simulink model "gm_sampleModel1839_4_sub"  (R2023a)
settings: Solver=VariableStepAuto  StartTime=0.0  StopTime=10.0  RelTol=1e-3
libraries: simulink x1
settings Model: Creator=user1  LastModifiedBy=user1
settings OptimizationCC: BlockReduction=off  ConditionallyExecuteInputs=off
settings DebuggingCC: InheritedTsInSrcMsg=none

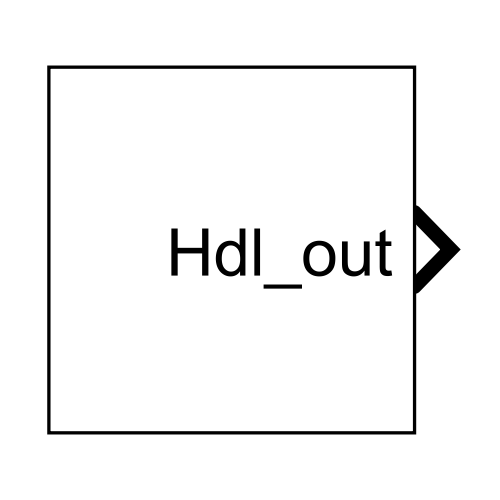
[thumbnail: Simulink's stored preview of the top-level diagram]
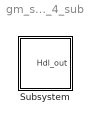
== system gm_sampleModel1839_4_sub ==
  Subsystem : Subsystem

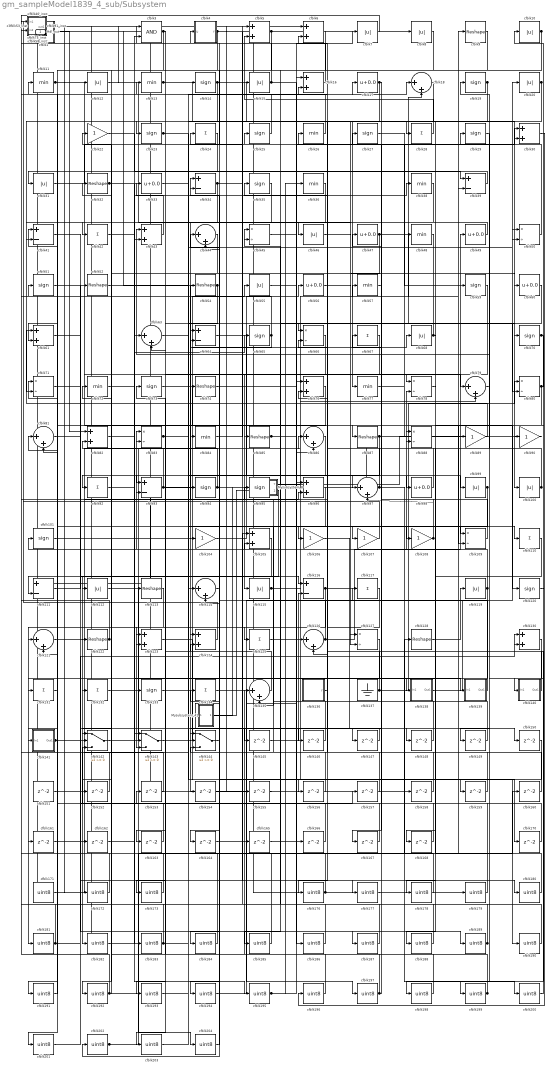
== system gm_sampleModel1839_4_sub/Subsystem ==
  Mysubsystem_41 : Subsystem
  Mysubsystem_8 : Subsystem
  cfblk1 : Subsystem  mask(Detect Rise Positive){vinit=double(0), InputProcessing=Elements as channels (sample based), OutDataTypeStr=uint8}
      mask prompts: vinit "Simulink:masks:InitialCondition_MP"; InputProcessing "Simulink:masks:InputProcessing_MP"; OutDataTypeStr "Simulink:masks:OutputDataType_MP"
      mask help: Simulink:masks:DetectRisePositive_MD
      mask init:
      | InputProcessing = 'Elements as channels (sample based)';
      | OutDataTypeStr = 'uint8';
      | vinit = double(0);
      mask TypeOptions InputProcessing: Simulink:masks:ColumnsAsChannelsFrameBased | Simulink:masks:ElementsAsChannelsSampleBased
      mask TypeOptions OutDataTypeStr: Simulink:masks:uint8 | Simulink:masks:boolean
      mask Display: fprintf('U > 0\n&  NOT\nU/z > 0')
  cfblk{7..8,10,12,15,20,31,46,55,68,99..100,112,115,119} (15 alike) : Abs  OutDataTypeStr=uint8  SaturateOnIntegerOverflow=off
  cfblk{14,19,23,25,27,29,35,51,59,65,70,73,94..95,101,120,133} (17 alike) : Signum
  cfblk102_inst : Subsystem
  cfblk{22,89..90,104,106..108} (7 alike) : Gain  OutDataTypeStr=uint8
  cfblk{5..6,16,30,43,61,76,82,96,105,123..124,130} (13 alike) : Sum  OutDataTypeStr=uint8
  cfblk{45,50,66,71,78,80,83,88,109,127} (10 alike) : Product  Inputs=*/  OutDataTypeStr=uint8  RndMeth=Zero  SaturateOnIntegerOverflow=on
  cfblk{11,13,26,36,38,48,57,72,77,84} (10 alike) : MinMax  OutDataTypeStr=uint8
  cfblk{24,28,42,67,92,110,117,125,131..132,134} (11 alike) : Sum  Inputs=+  OutDataTypeStr=uint8
  cfblk{34,39,41,64,93,111,116} (7 alike) : Sum  Inputs=+-  OutDataTypeStr=uint8
  cfblk{9,32,52,54,74,85,87,113,122,128} (10 alike) : Reshape
  cfblk{18,44,63,79,81,86,97,114,121,126,135} (11 alike) : Sum  Inputs=|++  OutDataTypeStr=uint8
  cfblk118_inst : Subsystem
  cfblk129_inst : Subsystem
  cfblk136 : Subsystem  mask(Counter Free-Running){NumBits=double(16), tsamp=double(-1)}
      mask prompts: NumBits "Simulink:masks:NumberOfBits_MP"; tsamp "Simulink:masks:SampleTime_MP"
      mask help: Simulink:masks:CounterFreeRunning_MD
  cfblk137 : Ground
  cfblk138 : Subsystem
  cfblk139 : Subsystem
  cfblk140 : Subsystem
  cfblk141 : Subsystem
  cfblk142 : Switch  OutDataTypeStr=uint8  SaturateOnIntegerOverflow=off  InputSameDT=off
  cfblk143 : Switch  OutDataTypeStr=uint8  SaturateOnIntegerOverflow=off  InputSameDT=off
  cfblk144 : Switch  OutDataTypeStr=uint8  SaturateOnIntegerOverflow=off  InputSameDT=off
  cfblk{145..168,170} (25 alike) : Delay  SampleTime=1
  cfblk{17,33,47,49,56,60,98} (7 alike) : Bias  Bias=0.0  SaturateOnIntegerOverflow=off
  cfblk{171..173,176..204} (32 alike) : DataTypeConversion  OutDataTypeStr=uint8  SaturateOnIntegerOverflow=off  RndMeth=Floor
  cfblk21_inst : Subsystem
  cfblk3 : Logic  AllPortsSameDT=off  OutDataTypeStr=boolean
  cfblk37_inst : Subsystem
  cfblk4 : Subsystem  mask(Detect Rise Nonnegative){vinit=double(0), InputProcessing=Elements as channels (sample based), OutDataTypeStr=uint8}
      mask prompts: vinit "Simulink:masks:InitialCondition_MP"; InputProcessing "Simulink:masks:InputProcessing_MP"; OutDataTypeStr "Simulink:masks:OutputDataType_MP"
      mask help: Simulink:masks:DetectRiseNonnegative_MD
      mask init:
      | InputProcessing = 'Elements as channels (sample based)';
      | OutDataTypeStr = 'uint8';
      | vinit = double(0);
      mask TypeOptions InputProcessing: Simulink:masks:ColumnsAsChannelsFrameBased | Simulink:masks:ElementsAsChannelsSampleBased
      mask TypeOptions OutDataTypeStr: Simulink:masks:uint8 | Simulink:masks:boolean
      mask Display: fprintf('U >= 0\n&  NOT\nU/z >= 0')
  cfblk40_inst : Subsystem
  cfblk53_inst : Subsystem
  cfblk58_inst : Subsystem
  cfblk75_inst : Subsystem
  cfblk91_inst : Subsystem
  Hdl_out : Outport  OutDataTypeStr=uint8  SampleTime=1
  wires:
  Mysubsystem_41/1(Out1) -> Mysubsystem_8/2(In2)
  Mysubsystem_8/1(Y) -> cfblk79/2
  Mysubsystem_8/2(Out2) -> cfblk111/2
  cfblk1/1(Y) -> cfblk82/1
  cfblk10/1 -> cfblk63/2, cfblk201/1
  cfblk100/1 -> cfblk43/1, cfblk16/2
  cfblk101/1 -> cfblk107/1
  cfblk102_inst/1(out1) -> cfblk6/1
  cfblk104/1 -> cfblk56/1
  cfblk105/1 -> cfblk182/1
  cfblk106/1 -> cfblk148/1
  cfblk107/1 -> cfblk102_inst/1(in1)
  cfblk108/1 -> cfblk97/2, cfblk24/1
  cfblk109/1 -> cfblk25/1
  cfblk11/1 -> cfblk115/1, cfblk78/1
  cfblk110/1 -> cfblk156/1
  cfblk111/1 -> cfblk52/1
  cfblk112/1 -> cfblk204/1
  cfblk113/1 -> cfblk181/1
  cfblk114/1 -> cfblk202/1
  cfblk115/1 -> cfblk18/2, cfblk170/1
  cfblk116/1 -> cfblk49/1, cfblk143/3
  cfblk117/1 -> cfblk176/1
  cfblk118_inst/1(out1) -> cfblk171/1
  cfblk119/1 -> cfblk83/1, cfblk161/1
  cfblk12/1 -> cfblk154/1
  cfblk120/1 -> cfblk198/1
  cfblk121/1 -> cfblk96/2
  cfblk122/1 -> cfblk41/1, cfblk129_inst/1(in1)
  cfblk123/1 -> cfblk190/1
  cfblk124/1 -> cfblk75_inst/2(in2)
  cfblk125/1 -> cfblk166/1
  cfblk126/1 -> cfblk101/1, cfblk78/2
  cfblk127/1 -> cfblk163/1
  cfblk128/1 -> cfblk119/1
  cfblk129_inst/1(out1) -> cfblk179/1, cfblk12/1
  cfblk13/1 -> cfblk100/1, cfblk127/2
  cfblk130/1 -> cfblk199/1
  cfblk131/1 -> cfblk71/1
  cfblk132/1 -> cfblk63/1
  cfblk133/1 -> cfblk55/1
  cfblk134/1 -> cfblk197/1
  cfblk135/1 -> cfblk73/1
  cfblk136/1(y) -> cfblk26/1
  cfblk137/1 -> cfblk95/1, cfblk80/1
  cfblk138/1(Out1) -> cfblk20/1
  cfblk139/1(Out1) -> cfblk51/1
  cfblk14/1 -> cfblk23/1, cfblk77/1
  cfblk140/1(Out1) -> cfblk35/1
  cfblk141/1(Out1) -> cfblk54/1, cfblk57/1
  cfblk142/1 -> cfblk9/1
  cfblk143/1 -> cfblk68/1
  cfblk144/1 -> cfblk34/1
  cfblk145/1 -> cfblk116/2
  cfblk146/1 -> cfblk64/1
  cfblk147/1 -> cfblk144/2
  cfblk148/1 -> cfblk66/2
  cfblk149/1 -> cfblk102_inst/2(in2)
  cfblk15/1 -> cfblk99/1, cfblk53_inst/2(in2)
  cfblk150/1 -> cfblk184/1
  cfblk151/1 -> cfblk96/1
  cfblk152/1 -> cfblk121/2
  cfblk153/1 -> cfblk37_inst/1(in1)
  cfblk154/1 -> cfblk50/2
  cfblk155/1 -> cfblk1/1(U)
  cfblk156/1 -> cfblk34/2
  cfblk157/1 -> cfblk76/2
  cfblk158/1 -> cfblk105/2
  cfblk159/1 -> cfblk126/2
  cfblk16/1 -> cfblk3/1
  cfblk160/1 -> cfblk6/2
  cfblk161/1 -> cfblk3/2
  cfblk162/1 -> cfblk143/1
  cfblk163/1 -> cfblk142/3
  cfblk164/1 -> cfblk135/1
  cfblk165/1 -> cfblk30/1
  cfblk166/1 -> cfblk82/2
  cfblk167/1 -> cfblk142/2
  cfblk168/1 -> cfblk144/3
  cfblk17/1 -> cfblk147/1, cfblk146/1
  cfblk170/1 -> cfblk11/1
  cfblk171/1 -> cfblk94/1
  cfblk172/1 -> cfblk118_inst/1(in1)
  cfblk173/1 -> cfblk118_inst/2(in2)
  cfblk176/1 -> cfblk58_inst/2(in2), cfblk44/1
  cfblk177/1 -> cfblk117/1
  cfblk178/1 -> cfblk153/1
  cfblk179/1 -> cfblk88/1
  cfblk18/1 -> cfblk124/1
  cfblk180/1 -> cfblk88/2
  cfblk181/1 -> cfblk91_inst/1(in1), cfblk187/1, cfblk157/1
  cfblk182/1 -> cfblk113/1
  cfblk183/1 -> cfblk53_inst/1(in1), cfblk50/1
  cfblk184/1 -> cfblk21_inst/1(in1)
  cfblk185/1 -> cfblk21_inst/2(in2)
  cfblk186/1 -> cfblk37_inst/2(in2)
  cfblk187/1 -> cfblk45/1
  cfblk188/1 -> cfblk45/2
  cfblk189/1 -> cfblk129_inst/2(in2), cfblk105/1
  cfblk19/1 -> cfblk194/1, cfblk84/1
  cfblk190/1 -> cfblk81/1
  cfblk191/1 -> cfblk81/2
  cfblk192/1 -> cfblk40_inst/2(in2), cfblk39/2, cfblk22/1
  cfblk193/1 -> cfblk86/1
  cfblk194/1 -> cfblk86/2
  cfblk195/1 -> cfblk76/1, cfblk36/1
  cfblk196/1 -> cfblk72/1
  cfblk197/1 -> cfblk47/1, cfblk124/2
  cfblk198/1 -> cfblk134/1
  cfblk199/1 -> cfblk93/2, cfblk155/1
  cfblk20/1 -> cfblk188/1, cfblk71/2, cfblk141/1(In1)
  cfblk200/1 -> cfblk130/1
  cfblk201/1 -> cfblk130/2
  cfblk202/1 -> cfblk128/1, cfblk160/1
  cfblk203/1 -> cfblk114/1
  cfblk204/1 -> cfblk114/2
  cfblk21_inst/1(out1) -> cfblk183/1
  cfblk22/1 -> cfblk39/1
  cfblk23/1 -> cfblk109/1, cfblk28/1
  cfblk24/1 -> cfblk112/1
  cfblk25/1 -> cfblk13/1
  cfblk26/1 -> cfblk58_inst/1(in1)
  cfblk27/1 -> cfblk59/1
  cfblk28/1 -> cfblk5/2
  cfblk29/1 -> cfblk149/1
  cfblk3/1 -> cfblk61/2, cfblk203/1
  cfblk30/1 -> cfblk196/1
  cfblk31/1 -> cfblk15/1
  cfblk32/1 -> cfblk43/2, cfblk127/1
  cfblk33/1 -> cfblk97/1
  cfblk34/1 -> cfblk79/1, cfblk193/1, cfblk143/2
  cfblk35/1 -> cfblk131/1
  cfblk36/1 -> cfblk41/2
  cfblk37_inst/1(out1) -> cfblk8/1, cfblk133/1
  cfblk38/1 -> cfblk132/1
  cfblk39/1 -> cfblk31/1
  cfblk4/1(Y) -> cfblk180/1, cfblk173/1, cfblk92/1, cfblk42/1
  cfblk40_inst/1(out1) -> cfblk75_inst/1(in1)
  cfblk41/1 -> cfblk150/1
  cfblk42/1 -> cfblk38/1
  cfblk43/1 -> cfblk33/1
  cfblk44/1 -> cfblk93/1
  cfblk45/1 -> cfblk186/1
  cfblk46/1 -> cfblk60/1
  cfblk47/1 -> cfblk80/2, cfblk152/1
  cfblk48/1 -> cfblk125/1
  cfblk49/1 -> cfblk46/1
  cfblk5/1 -> cfblk165/1, cfblk164/1
  cfblk50/1 -> cfblk4/1(U)
  cfblk51/1 -> cfblk116/1
  cfblk52/1 -> cfblk70/1
  cfblk53_inst/1(out1) -> cfblk172/1
  cfblk54/1 -> cfblk123/2, Hdl_out/1
  cfblk55/1 -> cfblk7/1
  cfblk56/1 -> cfblk98/1
  cfblk57/1 -> cfblk167/1
  cfblk58_inst/1(out1) -> cfblk14/1
  cfblk59/1 -> cfblk123/1
  cfblk6/1 -> cfblk144/1
  cfblk60/1 -> cfblk145/1
  cfblk61/1 -> cfblk162/1
  cfblk63/1 -> cfblk18/1
  cfblk64/1 -> cfblk126/1
  cfblk65/1 -> cfblk91_inst/2(in2), cfblk64/2
  cfblk66/1 -> cfblk85/1
  cfblk67/1 -> cfblk106/1
  cfblk68/1 -> cfblk66/1, cfblk168/1
  cfblk7/1 -> cfblk40_inst/1(in1)
  cfblk70/1 -> cfblk90/1, cfblk140/1(In1)
  cfblk71/1 -> cfblk177/1
  cfblk72/1 -> cfblk195/1
  cfblk73/1 -> cfblk120/1
  cfblk74/1 -> cfblk27/1
  cfblk75_inst/1(out1) -> cfblk151/1
  cfblk76/1 -> cfblk121/1
  cfblk77/1 -> cfblk48/1
  cfblk78/1 -> cfblk108/1
  cfblk79/1 -> cfblk19/1
  cfblk8/1 -> cfblk122/1
  cfblk80/1 -> cfblk10/1, cfblk109/2, cfblk138/1(In1)
  cfblk81/1 -> cfblk189/1
  cfblk82/1 -> cfblk65/1
  cfblk83/1 -> cfblk74/1, cfblk159/1
  cfblk84/1 -> cfblk5/1
  cfblk85/1 -> cfblk87/1, cfblk17/1
  cfblk86/1 -> cfblk192/1
  cfblk87/1 -> cfblk30/2, cfblk29/1, cfblk104/1
  cfblk88/1 -> cfblk178/1
  cfblk89/1 -> cfblk61/1
  cfblk9/1 -> cfblk185/1
  cfblk90/1 -> Mysubsystem_8/1(In1)
  cfblk91_inst/1(out1) -> cfblk158/1
  cfblk92/1 -> cfblk139/1(In1)
  cfblk93/1 -> cfblk83/2, cfblk110/1
  cfblk94/1 -> cfblk44/2, cfblk32/1
  cfblk95/1 -> cfblk111/1, cfblk89/1, Mysubsystem_41/1(In1)
  cfblk96/1 -> cfblk135/2
  cfblk97/1 -> cfblk200/1, cfblk16/1
  cfblk98/1 -> cfblk67/1
  cfblk99/1 -> cfblk191/1, cfblk142/1

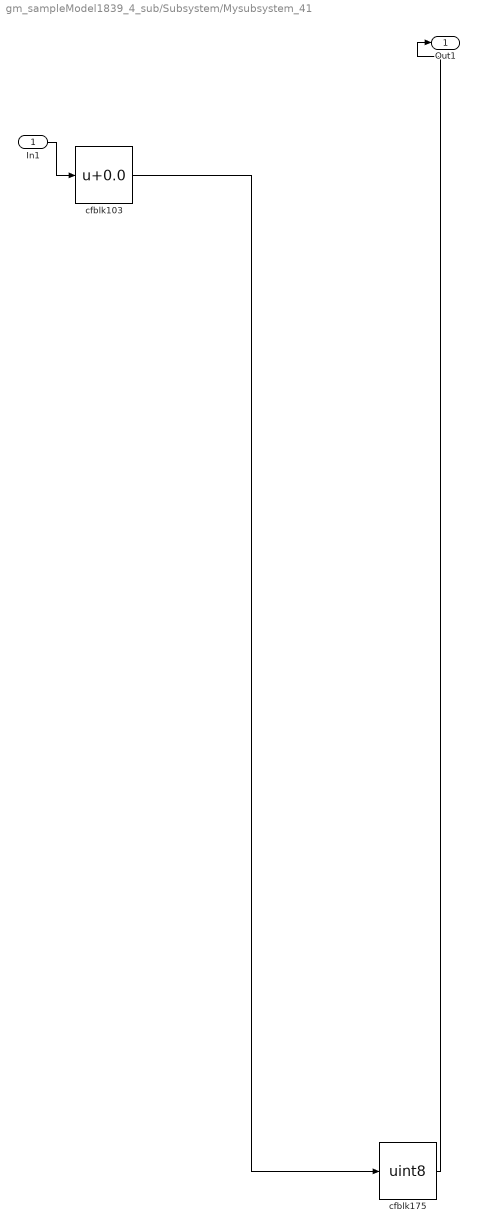
== system gm_sampleModel1839_4_sub/Subsystem/Mysubsystem_41 ==
  In1 : Inport  OutDataTypeStr=uint8  PortDimensions=1  SampleTime=1
  cfblk103 : Bias  Bias=0.0  SaturateOnIntegerOverflow=off
  cfblk175 : DataTypeConversion  OutDataTypeStr=uint8  SaturateOnIntegerOverflow=off  RndMeth=Floor
  Out1 : Outport  SampleTime=1
  wires:
  In1/1 -> cfblk103/1
  cfblk103/1 -> cfblk175/1
  cfblk175/1 -> Out1/1

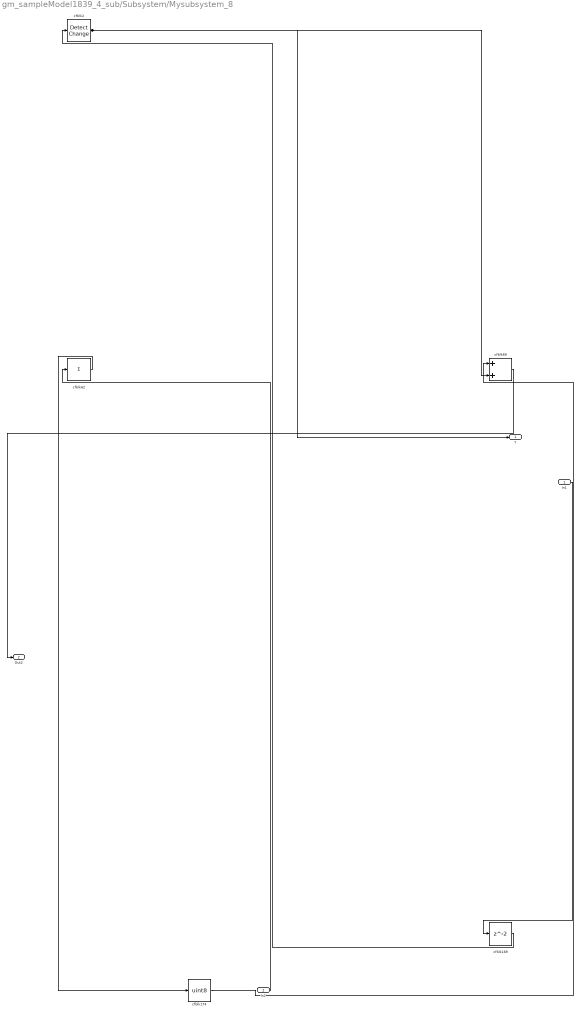
== system gm_sampleModel1839_4_sub/Subsystem/Mysubsystem_8 ==
  In1 : Inport  OutDataTypeStr=uint8  PortDimensions=1  SampleTime=1
  In2 : Inport  Port=2  OutDataTypeStr=uint8  PortDimensions=1  SampleTime=1
  cfblk169 : Delay  SampleTime=1
  cfblk174 : DataTypeConversion  OutDataTypeStr=uint8  SaturateOnIntegerOverflow=off  RndMeth=Floor
  cfblk2 : simulink/Logic and Bit Operations/Detect Change  vinit=0  OutDataTypeStr=boolean
      settings: LibrarySourceBlock=|
      | hdlsllib/Logic and Bit
      | Operations/Detect
      | Change
  cfblk62 : Sum  Inputs=+
  cfblk69 : Sum
  Y : Outport  SampleTime=1
  Out2 : Outport  Port=2  SampleTime=1
  wires:
  In1/1 -> cfblk169/1
  In2/1 -> cfblk62/1
  cfblk169/1 -> cfblk2/1
  cfblk174/1 -> cfblk69/1
  cfblk2/1 -> cfblk69/2, Y/1
  cfblk62/1 -> cfblk174/1
  cfblk69/1 -> Out2/1

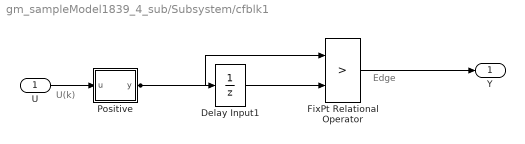
== system gm_sampleModel1839_4_sub/Subsystem/cfblk1 ==
  note: U(k)
  note: Edge
  U : Inport  OutDataTypeStr=uint8  SampleTime=1
  Delay Input1 : UnitDelay  Description=Store in Global RAM  DisableCoverage=on  InitialCondition=vinit  SampleTime=-1  HasFrameUpgradeWarning=on
  FixPt Relational Operator : RelationalOperator  Operator=>  OutDataTypeStr=fixdt(0, 8)  ZeroCross=off  InputSameDT=off
  Positive : Subsystem  mask(Compare To Zero){relop=>, OutDataTypeStr=boolean, ZeroCross=off}
      mask prompts: relop "Simulink:masks:Operator_MP"; OutDataTypeStr "Simulink:masks:OutputDataType_MP"; ZeroCross "Simulink:masks:EnableZerocrossingDetection_MP"
      mask help: Simulink:masks:CompareToZero_MD
      mask init:
      | OutDataTypeStr = 'boolean';
      | ZeroCross = 'off';
      | blkName = 'sampleModel1839_4_sub/Subsystem/cfblk1/Positive';
      | relop = '>';
      | setValue = 'boolean';
      mask TypeOptions relop: == | ~= | < | <= | >= | >
      mask TypeOptions OutDataTypeStr: Simulink:masks:uint8 | Simulink:masks:boolean
      mask Callback ZeroCross: sl('zeroCrossEnable', gcbh);
      mask Display: disp([relop,' 0'])
  Y : Outport  SampleTime=1
  wires:
  U/1 -> Positive/1(u)
  Delay Input1/1 -> FixPt Relational Operator/2
  FixPt Relational Operator/1 -> Y/1
  Positive/1(y) -> FixPt Relational Operator/1, Delay Input1/1

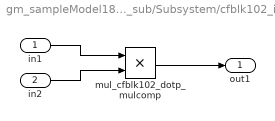
== system gm_sampleModel1839_4_sub/Subsystem/cfblk102_inst ==
  in1 : Inport  OutDataTypeStr=uint8  SampleTime=1
  in2 : Inport  Port=2  OutDataTypeStr=uint8  SampleTime=1
  mul_cfblk102_dotp_mulcomp : Product  Inputs=**  OutDataTypeStr=uint8  SampleTime=1
  out1 : Outport  OutDataTypeStr=uint8  SampleTime=1
  wires:
  in1/1 -> mul_cfblk102_dotp_mulcomp/1
  in2/1 -> mul_cfblk102_dotp_mulcomp/2
  mul_cfblk102_dotp_mulcomp/1 -> out1/1

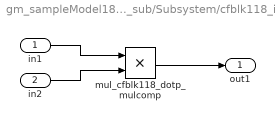
== system gm_sampleModel1839_4_sub/Subsystem/cfblk118_inst ==
  in1 : Inport  OutDataTypeStr=uint8  SampleTime=1
  in2 : Inport  Port=2  OutDataTypeStr=uint8  SampleTime=1
  mul_cfblk118_dotp_mulcomp : Product  Inputs=**  OutDataTypeStr=uint8  SampleTime=1
  out1 : Outport  OutDataTypeStr=uint8  SampleTime=1
  wires:
  in1/1 -> mul_cfblk118_dotp_mulcomp/1
  in2/1 -> mul_cfblk118_dotp_mulcomp/2
  mul_cfblk118_dotp_mulcomp/1 -> out1/1

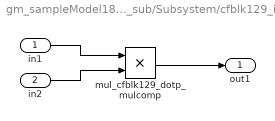
== system gm_sampleModel1839_4_sub/Subsystem/cfblk129_inst ==
  in1 : Inport  OutDataTypeStr=uint8  SampleTime=1
  in2 : Inport  Port=2  OutDataTypeStr=uint8  SampleTime=1
  mul_cfblk129_dotp_mulcomp : Product  Inputs=**  OutDataTypeStr=uint8  SampleTime=1
  out1 : Outport  OutDataTypeStr=uint8  SampleTime=1
  wires:
  in1/1 -> mul_cfblk129_dotp_mulcomp/1
  in2/1 -> mul_cfblk129_dotp_mulcomp/2
  mul_cfblk129_dotp_mulcomp/1 -> out1/1

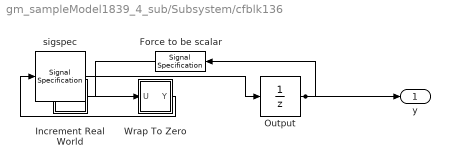
== system gm_sampleModel1839_4_sub/Subsystem/cfblk136 ==
  Force to be scalar : SignalSpecification  DisableCoverage=on  Dimensions=1
  Increment Real World : Subsystem  mask(Real World Value Increment){}
      mask help: Simulink:masks:RealWorldValueIncrement_MD
      mask Display: disp('V++')
  Output : UnitDelay  InitialCondition=0.0  SampleTime=tsamp  HasFrameUpgradeWarning=on
  Wrap To Zero : Subsystem  mask(Wrap To Zero){Threshold=double(65535)}
      mask prompts: Threshold "Simulink:masks:Threshold_MP"
      mask help: Simulink:masks:WrapToZero_MD
  sigspec : SignalSpecification  OutDataTypeStr=uint16  Dimensions=1
  y : Outport  SampleTime=1
  wires:
  Force to be scalar/1 -> Increment Real World/1(u)
  Increment Real World/1(y) -> Wrap To Zero/1(U)
  Output/1 -> Force to be scalar/1, y/1
  Wrap To Zero/1(Y) -> sigspec/1
  sigspec/1 -> Output/1

== system gm_sampleModel1839_4_sub/Subsystem/cfblk138 ==
  In1 : Inport  OutDataTypeStr=uint8  PortDimensions=1  SampleTime=1
  Out1 : Outport  SampleTime=1
  wires:
  In1/1 -> Out1/1

== system gm_sampleModel1839_4_sub/Subsystem/cfblk139 ==
  In1 : Inport  OutDataTypeStr=uint8  PortDimensions=1  SampleTime=1
  Out1 : Outport  SampleTime=1
  wires:
  In1/1 -> Out1/1

== system gm_sampleModel1839_4_sub/Subsystem/cfblk140 ==
  In1 : Inport  OutDataTypeStr=uint8  PortDimensions=1  SampleTime=1
  Out1 : Outport  SampleTime=1
  wires:
  In1/1 -> Out1/1

== system gm_sampleModel1839_4_sub/Subsystem/cfblk141 ==
  In1 : Inport  OutDataTypeStr=uint8  PortDimensions=1  SampleTime=1
  Out1 : Outport  SampleTime=1
  wires:
  In1/1 -> Out1/1

== system gm_sampleModel1839_4_sub/Subsystem/cfblk21_inst ==
  in1 : Inport  OutDataTypeStr=uint8  SampleTime=1
  in2 : Inport  Port=2  OutDataTypeStr=uint8  SampleTime=1
  mul_cfblk21_dotp_mulcomp : Product  Inputs=**  OutDataTypeStr=uint8  SampleTime=1
  out1 : Outport  OutDataTypeStr=uint8  SampleTime=1
  wires:
  in1/1 -> mul_cfblk21_dotp_mulcomp/1
  in2/1 -> mul_cfblk21_dotp_mulcomp/2
  mul_cfblk21_dotp_mulcomp/1 -> out1/1

== system gm_sampleModel1839_4_sub/Subsystem/cfblk37_inst ==
  in1 : Inport  OutDataTypeStr=uint8  SampleTime=1
  in2 : Inport  Port=2  OutDataTypeStr=uint8  SampleTime=1
  mul_cfblk37_dotp_mulcomp : Product  Inputs=**  OutDataTypeStr=uint8  SampleTime=1
  out1 : Outport  OutDataTypeStr=uint8  SampleTime=1
  wires:
  in1/1 -> mul_cfblk37_dotp_mulcomp/1
  in2/1 -> mul_cfblk37_dotp_mulcomp/2
  mul_cfblk37_dotp_mulcomp/1 -> out1/1

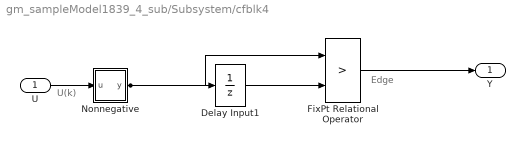
== system gm_sampleModel1839_4_sub/Subsystem/cfblk4 ==
  note: U(k)
  note: Edge
  U : Inport  OutDataTypeStr=uint8  SampleTime=1
  Delay Input1 : UnitDelay  Description=Store in Global RAM  DisableCoverage=on  InitialCondition=vinit  SampleTime=-1  HasFrameUpgradeWarning=on
  FixPt Relational Operator : RelationalOperator  Operator=>  OutDataTypeStr=fixdt(0, 8)  ZeroCross=off  InputSameDT=off
  Nonnegative : Subsystem  mask(Compare To Zero){relop=>=, OutDataTypeStr=boolean, ZeroCross=off}
      mask prompts: relop "Simulink:masks:Operator_MP"; OutDataTypeStr "Simulink:masks:OutputDataType_MP"; ZeroCross "Simulink:masks:EnableZerocrossingDetection_MP"
      mask help: Simulink:masks:CompareToZero_MD
      mask init:
      | OutDataTypeStr = 'boolean';
      | ZeroCross = 'off';
      | blkName = 'sampleModel1839_4_sub/Subsystem/cfblk4/Nonnegative';
      | relop = '>=';
      | setValue = 'boolean';
      mask TypeOptions relop: == | ~= | < | <= | >= | >
      mask TypeOptions OutDataTypeStr: Simulink:masks:uint8 | Simulink:masks:boolean
      mask Callback ZeroCross: sl('zeroCrossEnable', gcbh);
      mask Display: disp([relop,' 0'])
  Y : Outport  SampleTime=1
  wires:
  U/1 -> Nonnegative/1(u)
  Delay Input1/1 -> FixPt Relational Operator/2
  FixPt Relational Operator/1 -> Y/1
  Nonnegative/1(y) -> FixPt Relational Operator/1, Delay Input1/1

== system gm_sampleModel1839_4_sub/Subsystem/cfblk40_inst ==
  in1 : Inport  OutDataTypeStr=uint8  SampleTime=1
  in2 : Inport  Port=2  OutDataTypeStr=uint8  SampleTime=1
  mul_cfblk40_dotp_mulcomp : Product  Inputs=**  OutDataTypeStr=uint8  SampleTime=1
  out1 : Outport  OutDataTypeStr=uint8  SampleTime=1
  wires:
  in1/1 -> mul_cfblk40_dotp_mulcomp/1
  in2/1 -> mul_cfblk40_dotp_mulcomp/2
  mul_cfblk40_dotp_mulcomp/1 -> out1/1

== system gm_sampleModel1839_4_sub/Subsystem/cfblk53_inst ==
  in1 : Inport  OutDataTypeStr=uint8  SampleTime=1
  in2 : Inport  Port=2  OutDataTypeStr=uint8  SampleTime=1
  mul_cfblk53_dotp_mulcomp : Product  Inputs=**  OutDataTypeStr=uint8  SampleTime=1
  out1 : Outport  OutDataTypeStr=uint8  SampleTime=1
  wires:
  in1/1 -> mul_cfblk53_dotp_mulcomp/1
  in2/1 -> mul_cfblk53_dotp_mulcomp/2
  mul_cfblk53_dotp_mulcomp/1 -> out1/1

== system gm_sampleModel1839_4_sub/Subsystem/cfblk58_inst ==
  in1 : Inport  OutDataTypeStr=uint8  SampleTime=1
  in2 : Inport  Port=2  OutDataTypeStr=uint8  SampleTime=1
  mul_cfblk58_dotp_mulcomp : Product  Inputs=**  OutDataTypeStr=uint8  SampleTime=1
  out1 : Outport  OutDataTypeStr=uint8  SampleTime=1
  wires:
  in1/1 -> mul_cfblk58_dotp_mulcomp/1
  in2/1 -> mul_cfblk58_dotp_mulcomp/2
  mul_cfblk58_dotp_mulcomp/1 -> out1/1

== system gm_sampleModel1839_4_sub/Subsystem/cfblk75_inst ==
  in1 : Inport  OutDataTypeStr=uint8  SampleTime=1
  in2 : Inport  Port=2  OutDataTypeStr=uint8  SampleTime=1
  mul_cfblk75_dotp_mulcomp : Product  Inputs=**  OutDataTypeStr=uint8  SampleTime=1
  out1 : Outport  OutDataTypeStr=uint8  SampleTime=1
  wires:
  in1/1 -> mul_cfblk75_dotp_mulcomp/1
  in2/1 -> mul_cfblk75_dotp_mulcomp/2
  mul_cfblk75_dotp_mulcomp/1 -> out1/1

== system gm_sampleModel1839_4_sub/Subsystem/cfblk91_inst ==
  in1 : Inport  OutDataTypeStr=uint8  SampleTime=1
  in2 : Inport  Port=2  OutDataTypeStr=uint8  SampleTime=1
  mul_cfblk91_dotp_mulcomp : Product  Inputs=**  OutDataTypeStr=uint8  SampleTime=1
  out1 : Outport  OutDataTypeStr=uint8  SampleTime=1
  wires:
  in1/1 -> mul_cfblk91_dotp_mulcomp/1
  in2/1 -> mul_cfblk91_dotp_mulcomp/2
  mul_cfblk91_dotp_mulcomp/1 -> out1/1

== system gm_sampleModel1839_4_sub/Subsystem/cfblk1/Positive ==
  u : Inport  OutDataTypeStr=uint8  SampleTime=1
  Compare : RelationalOperator  Operator=>  OutDataTypeStr=boolean  ZeroCross=off
  Constant : Constant  DisableCoverage=on  Value=0  OutDataTypeStr=Inherit: Inherit via back propagation  SampleTime=-1  PreserveConstantTs=on
  y : Outport  SampleTime=1
  wires:
  u/1 -> Compare/1
  Compare/1 -> y/1
  Constant/1 -> Compare/2

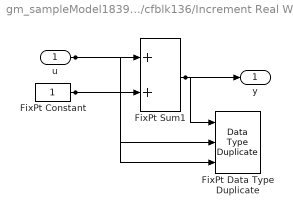
== system gm_sampleModel1839_4_sub/Subsystem/cfblk136/Increment Real World ==
  u : Inport  OutDataTypeStr=uint16  SampleTime=1
  FixPt Constant : Constant  DisableCoverage=on  OutDataTypeStr=Inherit: Inherit via back propagation  SampleTime=-1
  FixPt Data Type Duplicate : DataTypeDuplicate  DisableCoverage=on  NumInputPorts=3
  FixPt Sum1 : Sum  InputSameDT=on  OutDataTypeStr=Inherit: Inherit via back propagation  LockScale=on
  y : Outport  SampleTime=1
  wires:
  u/1 -> FixPt Sum1/1, FixPt Data Type Duplicate/2
  FixPt Constant/1 -> FixPt Sum1/2, FixPt Data Type Duplicate/3
  FixPt Sum1/1 -> FixPt Data Type Duplicate/1, y/1

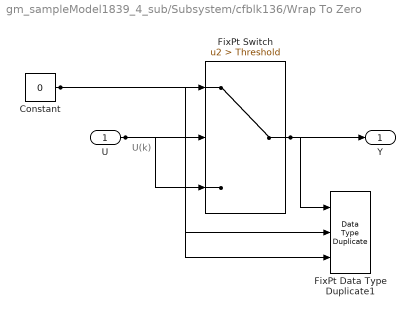
== system gm_sampleModel1839_4_sub/Subsystem/cfblk136/Wrap To Zero ==
  note: U(k)
  U : Inport  OutDataTypeStr=uint16  SampleTime=1
  Constant : Constant  DisableCoverage=on  Value=0  OutDataTypeStr=Inherit: Inherit via back propagation  SampleTime=-1
  FixPt Data Type Duplicate1 : DataTypeDuplicate  DisableCoverage=on  NumInputPorts=3
  FixPt Switch : Switch  Criteria=u2 > Threshold  Threshold=Threshold  OutDataTypeStr=Inherit: Inherit via back propagation  ZeroCross=off  SaturateOnIntegerOverflow=off  InputSameDT=off
  Y : Outport  SampleTime=1
  wires:
  U/1 -> FixPt Switch/3, FixPt Switch/2, FixPt Data Type Duplicate1/2
  Constant/1 -> FixPt Switch/1, FixPt Data Type Duplicate1/3
  FixPt Switch/1 -> FixPt Data Type Duplicate1/1, Y/1

== system gm_sampleModel1839_4_sub/Subsystem/cfblk4/Nonnegative ==
  u : Inport  OutDataTypeStr=uint8  SampleTime=1
  Compare : RelationalOperator  OutDataTypeStr=boolean  ZeroCross=off
  Constant : Constant  DisableCoverage=on  Value=0  OutDataTypeStr=Inherit: Inherit via back propagation  SampleTime=-1  PreserveConstantTs=on
  y : Outport  SampleTime=1
  wires:
  u/1 -> Compare/1
  Compare/1 -> y/1
  Constant/1 -> Compare/2
